simulink model "Sistarref"  (Simulink 7.5)
settings: Solver=ode3  StartTime=0.0  StopTime=25.0  RelTol=1e-3
values from neighbouring files (symbols this model uses):
  g = 9.81    [InitialParameters.m]
  m = 825    [InitialParameters.m]
  M1 = 4.273    [InitialParameters.m]
  M2 = 2.238    [InitialParameters.m]
  Md = 4.067    [InitialParameters.m]
  Ni = 0.94    [InitialParameters.m]
  rd = 0.274    [InitialParameters.m]
  ro = 0.752    [InitialParameters.m]
undefined symbols (not defined in the file or in its folder): b0, b2, Cx, senalfa2, Sf, t0, t00, t1, t11, V1
settings Model: Creator=user  LastModifiedBy=user
settings DebuggingCC: StrictBusMsg=Warning

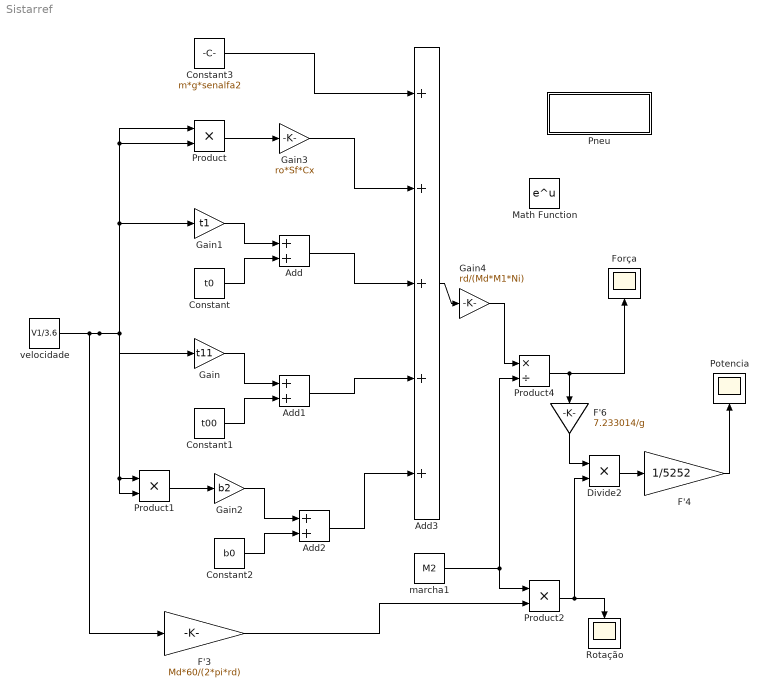
== system Sistarref ==
  Add : Sum  OutDataType=fixdt(1, 16)  OutScaling=2^-10
  Add1 : Sum  OutDataType=fixdt(1, 16)  OutScaling=2^-10
  Add2 : Sum  OutDataType=fixdt(1, 16)  OutScaling=2^-10
  Add3 : Sum  Inputs=+++++  OutDataType=fixdt(1, 16)  OutScaling=2^-10
  Constant : Constant  Value=t0  OutDataType=fixdt(1, 16)  OutScaling=2^0
  Constant1 : Constant  Value=t00  OutDataType=fixdt(1, 16)  OutScaling=2^0
  Constant2 : Constant  Value=b0  OutDataType=fixdt(1, 16)  OutScaling=2^0
  Constant3 : Constant  Value=m*g*senalfa2  OutDataType=fixdt(1, 16)  OutScaling=2^0
  Divide2 : Product  Inputs=**  OutDataType=fixdt(1, 16)  OutScaling=2^-10
  F'3 : Gain  Gain=Md*60/(2*pi*rd)  ParameterDataType=fixdt(1, 16)  ParameterScaling=2^0  OutDataType=fixdt(1, 16)  OutScaling=2^0
  F'4 : Gain  Gain=1/5252  ParameterDataType=fixdt(1, 16)  ParameterScaling=2^0  OutDataType=fixdt(1, 16)  OutScaling=2^0
  F'6 : Gain  Gain=7.233014/g  ParameterDataType=fixdt(1, 16)  ParameterScaling=2^0  OutDataType=fixdt(1, 16)  OutScaling=2^0
  Força : Scope
  Gain : Gain  Gain=t11  ParameterDataType=fixdt(1, 16)  ParameterScaling=2^0  OutDataType=fixdt(1, 16)  OutScaling=2^0
  Gain1 : Gain  Gain=t1  ParameterDataType=fixdt(1, 16)  ParameterScaling=2^0  OutDataType=fixdt(1, 16)  OutScaling=2^0
  Gain2 : Gain  Gain=b2  ParameterDataType=fixdt(1, 16)  ParameterScaling=2^0  OutDataType=fixdt(1, 16)  OutScaling=2^0
  Gain3 : Gain  Gain=ro*Sf*Cx  ParameterDataType=fixdt(1, 16)  ParameterScaling=2^0  OutDataType=fixdt(1, 16)  OutScaling=2^0
  Gain4 : Gain  Gain=rd/(Md*M1*Ni)  ParameterDataType=fixdt(1, 16)  ParameterScaling=2^0  OutDataType=fixdt(1, 16)  OutScaling=2^0
  Math Function : Math  OutDataType=fixdt(1, 16)  OutScaling=2^0  SaturateOnIntegerOverflow=on
  Pneu : Subsystem  TreatAsAtomicUnit=on
  Potencia : Scope
      settings: SaveName=ScopeData2
  Product : Product  OutDataType=fixdt(1, 16)  OutScaling=2^0  RndMeth=Zero
  Product1 : Product  OutDataType=fixdt(1, 16)  OutScaling=2^0  RndMeth=Zero
  Product2 : Product  OutDataType=fixdt(1, 16)  OutScaling=2^0  RndMeth=Zero
  Product4 : Product  Inputs=*/  OutDataType=fixdt(1, 16)  OutScaling=2^0  RndMeth=Zero
  Rotação : Scope
  marcha1 : Constant  Value=M2  OutDataType=fixdt(1, 16)  OutScaling=2^0
  velocidade : Constant  Value=V1/3.6  OutDataType=fixdt(1, 16)  OutScaling=2^0
  wires:
  Product/1 -> Gain3/1
  Constant1/1 -> Add1/2
  Gain/1 -> Add1/1
  Constant/1 -> Add/2
  Gain1/1 -> Add/1
  Add/1 -> Add3/3
  Add1/1 -> Add3/4
  Gain3/1 -> Add3/2
  Constant3/1 -> Add3/1
  Add3/1 -> Gain4/1
  Product1/1 -> Gain2/1
  Gain2/1 -> Add2/1
  Constant2/1 -> Add2/2
  Add2/1 -> Add3/5
  velocidade/1 -> Gain/1, Gain1/1, Product/2, Product/1, Product1/1, Product1/2, F'3/1
  Gain4/1 -> Product4/1
  marcha1/1 -> Product4/2, Product2/1
  F'3/1 -> Product2/2
  Product2/1 -> Rotação/1, Divide2/2
  Product4/1 -> Força/1, F'6/1
  Divide2/1 -> F'4/1
  F'6/1 -> Divide2/1
  F'4/1 -> Potencia/1

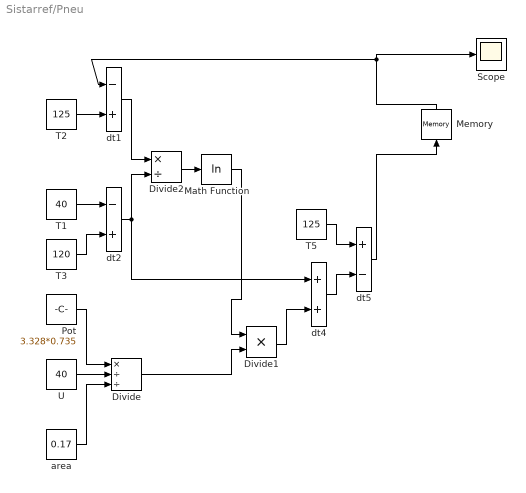
== system Sistarref/Pneu ==
  Divide : Product  Inputs=*//  OutDataType=fixdt(1, 16)  OutScaling=2^-10
  Divide1 : Product  Inputs=**  OutDataType=fixdt(1, 16)  OutScaling=2^-10
  Divide2 : Product  Inputs=*/  OutDataType=fixdt(1, 16)  OutScaling=2^-10
  Math Function : Math  Operator=log  OutDataType=fixdt(1, 16)  OutScaling=2^0  SaturateOnIntegerOverflow=on
  Memory : Memory  X0=60
  Pot : Constant  Value=3.328*0.735  OutDataType=fixdt(1, 16)  OutScaling=2^0
  Scope : Scope
      settings: SaveName=ScopeData3
  T1 : Constant  Value=40  OutDataType=fixdt(1, 16)  OutScaling=2^0
  T2 : Constant  Value=125  OutDataType=fixdt(1, 16)  OutScaling=2^0
  T3 : Constant  Value=120  OutDataType=fixdt(1, 16)  OutScaling=2^0
  T5 : Constant  Value=125  OutDataType=fixdt(1, 16)  OutScaling=2^0
  U : Constant  Value=40  OutDataType=fixdt(1, 16)  OutScaling=2^0
  area : Constant  Value=0.17  OutDataType=fixdt(1, 16)  OutScaling=2^0
  dt1 : Sum  Inputs=-+  OutDataType=fixdt(1, 16)  OutScaling=2^-10
  dt2 : Sum  Inputs=-+  OutDataType=fixdt(1, 16)  OutScaling=2^-10
  dt4 : Sum  OutDataType=fixdt(1, 16)  OutScaling=2^-10
  dt5 : Sum  Inputs=+-  OutDataType=fixdt(1, 16)  OutScaling=2^-10
  wires:
  T2/1 -> dt1/2
  T1/1 -> dt2/1
  T3/1 -> dt2/2
  area/1 -> Divide/3
  U/1 -> Divide/2
  Pot/1 -> Divide/1
  dt2/1 -> dt4/1, Divide2/2
  Divide/1 -> Divide1/2
  Math Function/1 -> Divide1/1
  Divide1/1 -> dt4/2
  dt4/1 -> dt5/2
  T5/1 -> dt5/1
  dt5/1 -> Memory/1
  Memory/1 -> dt1/1, Scope/1
  Divide2/1 -> Math Function/1
  dt1/1 -> Divide2/1
